simulink model "chap5_6sim"  (Simulink 7.7)
settings: Solver=ode45  StartTime=0.0  StopTime=100  FixedStep=0.001  RelTol=1e-3
libraries: simulink x1
settings Model: Creator=hp  LastModifiedBy=ljk  ExtModeTrigMode=oneshot  ExtModeArmWhenConnect=off
settings DataIOCC: LimitDataPoints=off  SignalLoggingName=sigsOut
settings OptimizationCC: BooleanDataType=off  InitFltsAndDblsToZero=on
settings DebuggingCC: SaveWithParameterizedLinksMsg=none  SignalResolutionControl=TryResolveAllWithWarning  SolverPrmCheckMsg=none  MultiTaskDSMMsg=warning  MultiTaskCondExecSysMsg=none  StrictBusMsg=None
settings HardwareCC: TargetUnknown=on
settings RTWCC: IncludeERTFirstTime=on
settings GRTTargetCC: TargetFcnLib=ansi_tfl_tmw.mat

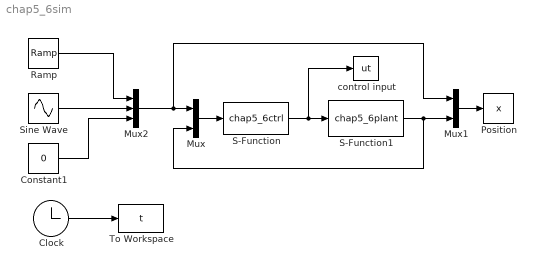
== system chap5_6sim ==
  Clock : Clock
      settings: Decimation=10
  Constant1 : Constant  Value=0
  Mux : Mux  Inputs=2
  Mux1 : Mux  Inputs=2
  Mux2 : Mux  Inputs=3
  Position : ToWorkspace  VariableName=x  SampleTime=-1  SaveFormat=Array
  Ramp : simulink/Sources/Ramp  SystemSampleTime=-1  slope=1  start=0  X0=0
  S-Function : S-Function  FunctionName=chap5_6ctrl  EnableBusSupport=off
  S-Function1 : S-Function  FunctionName=chap5_6plant  EnableBusSupport=off
  Sine Wave : Sin  SampleTime=0
  To Workspace : ToWorkspace  VariableName=t  SampleTime=-1  SaveFormat=Array
  control input : ToWorkspace  VariableName=ut  SampleTime=-1  SaveFormat=Array
  wires:
  S-Function/1 -> S-Function1/1, control input/1
  S-Function1/1 -> Mux1/2, Mux/2
  Clock/1 -> To Workspace/1
  Mux/1 -> S-Function/1
  Mux1/1 -> Position/1
  Mux2/1 -> Mux/1, Mux1/1
  Sine Wave/1 -> Mux2/2
  Constant1/1 -> Mux2/3
  Ramp/1 -> Mux2/1
